simulink model "Model_IPS7"  (R2016a)
settings: Solver=FixedStepAuto  StartTime=0  StopTime=2  FixedStep=1e-5
InitFcn:
  | parametriAM
values from neighbouring files (symbols this model uses):
  filtkonst = 1.3    [parametriAM.m]
  Imrn = 7.4    [parametriAM.m]
  In = 12.7    [parametriAM.m]
  Ismax = In*sqrt(2)    [parametriAM.m]
  J = 0.019    [parametriAM.m]
  Ki_Imr = 1000    [parametriAM.m]
  Ki_tok = 5.0    (= 5)    [parametriAM.m]
  Ki_wr = 1000    [parametriAM.m]
  Kp_Imr = 100    [parametriAM.m]
  Kp_tok = 0.05    [parametriAM.m]
  Kp_wr = 50    [parametriAM.m]
  Lm = 0.0493    [parametriAM.m]
  Lr = 0.05315    [parametriAM.m]
  Ls = 0.05315    [parametriAM.m]
  Lst = sigma*Ls    (= 0.00742111947319)    [parametriAM.m]
  pp = 3    [parametriAM.m]
  Rs = 0.594    [parametriAM.m]
  sigma = 1 - 1/((1+sigmaR)*(1+sigmaS))    (= 0.13962595434)    [parametriAM.m]
  Tr = Lr/Rr    (= 0.0771407837446)    [parametriAM.m]
  Udc = Un*sqrt(2)    [parametriAM.m]
  wb_upper_limit_field_weaking = sqrt((Ls^2+Lst^2)/(2*Lst^2*Ls^2))*Usmax/Ismax    [parametriAM.m]
  wdod = 2000*2*pi/60    (= 209.439510239)    [parametriAM.m]
libraries: simulink x18
(part 2 of 2)

== system Model_IPS7/Regulacija2/Transformacije/Inverzni Park ==
  kot : Inport
  U_dq : Inport  Port=2
  Demux : Demux  Outputs=2
  Mux : Mux  Inputs=2
  "Sum1 " : Sum  Inputs=+-  SaturateOnIntegerOverflow=on  InputSameDT=on  OutDataTypeStr=Inherit: Same as first input
  Sum2 : Sum  SaturateOnIntegerOverflow=on  InputSameDT=on  OutDataTypeStr=Inherit: Same as first input
  cos : Fcn  Expr=cos(u)
  sin : Fcn  Expr=sin(u)
  x_d*cos : Product  SaturateOnIntegerOverflow=on  RndMeth=Zero  InputSameDT=on  OutDataTypeStr=Inherit: Same as first input
  x_d*sin : Product  SaturateOnIntegerOverflow=on  RndMeth=Zero  InputSameDT=on  OutDataTypeStr=Inherit: Same as first input
  x_q*cos : Product  SaturateOnIntegerOverflow=on  RndMeth=Zero  InputSameDT=on  OutDataTypeStr=Inherit: Same as first input
  "x_q*sin " : Product  SaturateOnIntegerOverflow=on  RndMeth=Zero  InputSameDT=on  OutDataTypeStr=Inherit: Same as first input
  U_ab : Outport
  wires:
  Mux/1 -> U_ab/1
  U_dq/1 -> Demux/1
  Demux/1 -> x_d*sin/1, x_d*cos/1
  Demux/2 -> "x_q*sin "/1, x_q*cos/1
  cos/1 -> x_q*cos/2, x_d*cos/2
  sin/1 -> "x_q*sin "/2, x_d*sin/2
  x_d*cos/1 -> "Sum1 "/1
  "x_q*sin "/1 -> "Sum1 "/2
  x_q*cos/1 -> Sum2/2
  x_d*sin/1 -> Sum2/1
  "Sum1 "/1 -> Mux/1
  Sum2/1 -> Mux/2
  kot/1 -> cos/1, sin/1

== system Model_IPS7/Regulacija2/Transformacije/Park ==
  I_ab : Inport
  kot : Inport  Port=2
  Demux : Demux  Outputs=2
  Mux : Mux  Inputs=2
  "Sum1 " : Sum  SaturateOnIntegerOverflow=on  InputSameDT=on  OutDataTypeStr=Inherit: Same as first input
  Sum2 : Sum  Inputs=-+  SaturateOnIntegerOverflow=on  InputSameDT=on  OutDataTypeStr=Inherit: Same as first input
  cos : Fcn  Expr=cos(u)
  sin : Fcn  Expr=sin(u)
  x_a*cos : Product  SaturateOnIntegerOverflow=on  RndMeth=Zero  InputSameDT=on  OutDataTypeStr=Inherit: Same as first input
  x_a*sin : Product  SaturateOnIntegerOverflow=on  RndMeth=Zero  InputSameDT=on  OutDataTypeStr=Inherit: Same as first input
  x_b*cos : Product  SaturateOnIntegerOverflow=on  RndMeth=Zero  InputSameDT=on  OutDataTypeStr=Inherit: Same as first input
  "x_b*sin " : Product  SaturateOnIntegerOverflow=on  RndMeth=Zero  InputSameDT=on  OutDataTypeStr=Inherit: Same as first input
  I_dq : Outport
  wires:
  Mux/1 -> I_dq/1
  I_ab/1 -> Demux/1
  Demux/1 -> x_a*sin/1, x_a*cos/1
  Demux/2 -> "x_b*sin "/1, x_b*cos/1
  cos/1 -> x_b*cos/2, x_a*cos/2
  sin/1 -> "x_b*sin "/2, x_a*sin/2
  x_a*cos/1 -> "Sum1 "/1
  "x_b*sin "/1 -> "Sum1 "/2
  x_b*cos/1 -> Sum2/2
  x_a*sin/1 -> Sum2/1
  "Sum1 "/1 -> Mux/1
  Sum2/1 -> Mux/2
  kot/1 -> cos/1, sin/1

== system Model_IPS7/Regulacija1/Regulacija navora/Limita q toka/napetostna limita ==
  Iddej : Inport
  w : Inport  Port=2
  Abs : Abs
  Abs1 : Abs
  Add1 : Sum  Inputs=-+
  Constant : Constant
  Divide : Product  Inputs=*/
  Gain : Gain  Gain=-1
  Product2 : Product
  Product3 : Product
  Saturation : Saturate  UpperLimit=1  LowerLimit=0
  Sqrt : Sqrt  SaturateOnIntegerOverflow=on
  a : Subsystem
  b : Subsystem
  high : Outport
  low : Outport  Port=2
  wires:
  Sqrt/1 -> Product3/1
  Iddej/1 -> Divide/1
  Divide/1 -> Product2/1, Product2/2
  Constant/1 -> Add1/2
  w/1 -> Abs1/1
  Product3/1 -> Abs/1
  Add1/1 -> Sqrt/1
  b/1(b) -> Product3/2
  Gain/1 -> low/1
  a/1(a) -> Divide/2
  Abs/1 -> high/1, Gain/1
  Abs1/1 -> b/1(w), a/1(w)
  Product2/1 -> Saturation/1
  Saturation/1 -> Add1/1

== system Model_IPS7/Regulacija1/Regulacija navora/Limita q toka/tokovna ==
  Id : Inport
  Abs : Abs
  Constant : Constant  Value=Ismax^2
  Gain2 : Gain  Gain=-1
  Product1 : Product
  Saturation : Saturate  UpperLimit=Ismax*5  LowerLimit=0
  Sqrt : Sqrt  SaturateOnIntegerOverflow=on
  Subtract : Sum  Inputs=+-
  high : Outport
  low : Outport  Port=2
  wires:
  Sqrt/1 -> Abs/1
  Id/1 -> Product1/2, Product1/1
  Gain2/1 -> low/1
  Constant/1 -> Subtract/1
  Product1/1 -> Subtract/2
  Abs/1 -> high/1, Gain2/1
  Subtract/1 -> Saturation/1
  Saturation/1 -> Sqrt/1

== system Model_IPS7/Regulacija1/Transformacije/Clarke/ABC_ab1 ==
  A : Inport
  B : Inport  Port=2
  C : Inport  Port=3
  Gain1 : Gain  Gain=2
  Gain2 : Gain
  Gain24 : Gain  Gain=sqrt(3)/3
  Sum11 : Sum
  Terminator : Terminator
  alfa : Outport
  beta : Outport  Port=2
  wires:
  C/1 -> Terminator/1
  Gain1/1 -> Sum11/2
  B/1 -> Gain1/1
  Gain24/1 -> beta/1
  Gain2/1 -> alfa/1
  Sum11/1 -> Gain24/1
  A/1 -> Sum11/1, Gain2/1

== system Model_IPS7/Regulacija1/Transformacije/Inverzni Clarke/ab_ABC ==
  alfa : Inport
  beta : Inport  Port=2
  Gain1 : Gain
  Gain2 : Gain  Gain=-0.5
  Gain25 : Gain  Gain=sqrt(3)/2
  Gain3 : Gain  Gain=sqrt(3)/2
  Gain4 : Gain  Gain=0.5
  Sum10 : Sum
  Sum11 : Sum  Inputs=--
  A : Outport
  B : Outport  Port=2
  C : Outport  Port=3
  wires:
  Gain3/1 -> Sum11/2
  beta/1 -> Gain25/1, Gain3/1
  Gain4/1 -> Sum11/1
  Gain25/1 -> Sum10/2
  Gain2/1 -> Sum10/1
  alfa/1 -> Gain1/1, Gain2/1, Gain4/1
  Gain1/1 -> A/1
  Sum10/1 -> B/1
  Sum11/1 -> C/1

== system Model_IPS7/Regulacija2/Regulacija navora/Limita q toka/napetostna limita ==
  Iddej : Inport
  w : Inport  Port=2
  Abs : Abs
  Abs1 : Abs
  Add1 : Sum  Inputs=-+
  Constant : Constant
  Divide : Product  Inputs=*/
  Gain : Gain  Gain=-1
  Product2 : Product
  Product3 : Product
  Saturation : Saturate  UpperLimit=1  LowerLimit=0
  Sqrt : Sqrt  SaturateOnIntegerOverflow=on
  a : Subsystem
  b : Subsystem
  high : Outport
  low : Outport  Port=2
  wires:
  Sqrt/1 -> Product3/1
  Iddej/1 -> Divide/1
  Divide/1 -> Product2/1, Product2/2
  Constant/1 -> Add1/2
  w/1 -> Abs1/1
  Product3/1 -> Abs/1
  Add1/1 -> Sqrt/1
  b/1(b) -> Product3/2
  Gain/1 -> low/1
  a/1(a) -> Divide/2
  Abs/1 -> high/1, Gain/1
  Abs1/1 -> b/1(w), a/1(w)
  Product2/1 -> Saturation/1
  Saturation/1 -> Add1/1

== system Model_IPS7/Regulacija2/Regulacija navora/Limita q toka/tokovna ==
  Id : Inport
  Abs : Abs
  Constant : Constant  Value=Ismax^2
  Gain2 : Gain  Gain=-1
  Product1 : Product
  Saturation : Saturate  UpperLimit=Ismax*5  LowerLimit=0
  Sqrt : Sqrt  SaturateOnIntegerOverflow=on
  Subtract : Sum  Inputs=+-
  high : Outport
  low : Outport  Port=2
  wires:
  Sqrt/1 -> Abs/1
  Id/1 -> Product1/2, Product1/1
  Gain2/1 -> low/1
  Constant/1 -> Subtract/1
  Product1/1 -> Subtract/2
  Abs/1 -> high/1, Gain2/1
  Subtract/1 -> Saturation/1
  Saturation/1 -> Sqrt/1

== system Model_IPS7/Regulacija2/Transformacije/Clarke/ABC_ab1 ==
  A : Inport
  B : Inport  Port=2
  C : Inport  Port=3
  Gain1 : Gain  Gain=2
  Gain2 : Gain
  Gain24 : Gain  Gain=sqrt(3)/3
  Sum11 : Sum
  Terminator : Terminator
  alfa : Outport
  beta : Outport  Port=2
  wires:
  C/1 -> Terminator/1
  Gain1/1 -> Sum11/2
  B/1 -> Gain1/1
  Gain24/1 -> beta/1
  Gain2/1 -> alfa/1
  Sum11/1 -> Gain24/1
  A/1 -> Sum11/1, Gain2/1

== system Model_IPS7/Regulacija2/Transformacije/Inverzni Clarke/ab_ABC ==
  alfa : Inport
  beta : Inport  Port=2
  Gain1 : Gain
  Gain2 : Gain  Gain=-0.5
  Gain25 : Gain  Gain=sqrt(3)/2
  Gain3 : Gain  Gain=sqrt(3)/2
  Gain4 : Gain  Gain=0.5
  Sum10 : Sum
  Sum11 : Sum  Inputs=--
  A : Outport
  B : Outport  Port=2
  C : Outport  Port=3
  wires:
  Gain3/1 -> Sum11/2
  beta/1 -> Gain25/1, Gain3/1
  Gain4/1 -> Sum11/1
  Gain25/1 -> Sum10/2
  Gain2/1 -> Sum10/1
  alfa/1 -> Gain1/1, Gain2/1, Gain4/1
  Gain1/1 -> A/1
  Sum10/1 -> B/1
  Sum11/1 -> C/1

== system Model_IPS7/Regulacija1/Regulacija navora/Limita q toka/napetostna limita/a ==
  w : Inport
  Add3 : Sum
  Constant1 : Constant  Value=Udc/Ls
  Constant2 : Constant  Value=0.001
  Divide : Product  Inputs=*/
  a : Outport
  wires:
  Constant1/1 -> Divide/1
  Constant2/1 -> Add3/2
  Add3/1 -> Divide/2
  w/1 -> Add3/1
  Divide/1 -> a/1

== system Model_IPS7/Regulacija1/Regulacija navora/Limita q toka/napetostna limita/b ==
  w : Inport
  Add4 : Sum
  Constant3 : Constant  Value=Udc/Lst
  Constant4 : Constant  Value=0.001
  Divide1 : Product  Inputs=*/
  b : Outport
  wires:
  Divide1/1 -> b/1
  w/1 -> Add4/1
  Add4/1 -> Divide1/2
  Constant3/1 -> Divide1/1
  Constant4/1 -> Add4/2

== system Model_IPS7/Regulacija2/Regulacija navora/Limita q toka/napetostna limita/a ==
  w : Inport
  Add3 : Sum
  Constant1 : Constant  Value=Udc/Ls
  Constant2 : Constant  Value=0.001
  Divide : Product  Inputs=*/
  a : Outport
  wires:
  Constant1/1 -> Divide/1
  Constant2/1 -> Add3/2
  Add3/1 -> Divide/2
  w/1 -> Add3/1
  Divide/1 -> a/1

== system Model_IPS7/Regulacija2/Regulacija navora/Limita q toka/napetostna limita/b ==
  w : Inport
  Add4 : Sum
  Constant3 : Constant  Value=Udc/Lst
  Constant4 : Constant  Value=0.001
  Divide1 : Product  Inputs=*/
  b : Outport
  wires:
  Divide1/1 -> b/1
  w/1 -> Add4/1
  Add4/1 -> Divide1/2
  Constant3/1 -> Divide1/1
  Constant4/1 -> Add4/2
